simulink model "Modelo_termometro"  (R2020b)
settings: Solver=VariableStepAuto  StartTime=0.0  StopTime=5  RelTol=1e-3
settings Model: Creator=Marce  LastModifiedBy=Marce

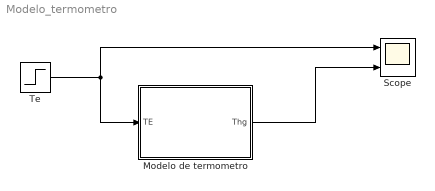
== system Modelo_termometro ==
  Modelo de termometro : Subsystem  mask{R1=0.1, R2=0.1, Cv=1, Chg=1}
      mask prompts: R1 "Resistencia térmica de convección aire/vidrio"; R2 "Resistencia térmica de convección vidrio/mercurio"; Cv "Capacidad Calorífica del Vidrio"; Chg "Capacidad Calorífica del Mercurio"
  Scope : Scope  NumInputPorts=2
  Te : Step  After=50  SampleTime=0
  wires:
  Te/1 -> Scope/1, Modelo de termometro/1(TE)
  Modelo de termometro/1(Thg) -> Scope/2

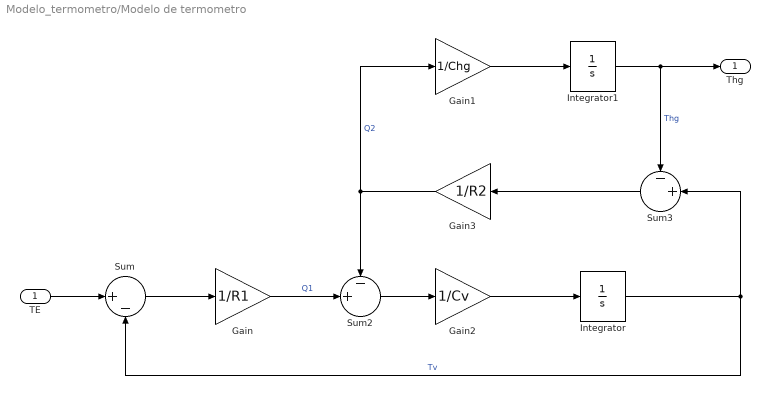
== system Modelo_termometro/Modelo de termometro ==
  TE : Inport
  Gain : Gain  Gain=1/R1
  Gain1 : Gain  Gain=1/Chg
  Gain2 : Gain  Gain=1/Cv
  Gain3 : Gain  Gain=1/R2
  Integrator : Integrator
  Integrator1 : Integrator
  Sum : Sum  Inputs=|+-
  Sum2 : Sum  Inputs=-+|
  Sum3 : Sum  Inputs=-+|
  Thg : Outport
  wires:
  TE/1 -> Sum/1
  Gain3/1 -> Gain1/1, Sum2/1  "Q2"
  Gain1/1 -> Integrator1/1
  Sum2/1 -> Gain2/1
  Gain2/1 -> Integrator/1
  Integrator1/1 -> Thg/1, Sum3/1  "Thg"
  Gain/1 -> Sum2/2  "Q1"
  Sum/1 -> Gain/1
  Integrator/1 -> Sum3/2, Sum/2  "Tv"
  Sum3/1 -> Gain3/1
